simulink model "pole_placement_with_disturbance"  (R2023b)
settings: Solver=FixedStepAuto  StartTime=0.0  StopTime=Tend_slk  RelTol=1e-3
values from neighbouring files (symbols this model uses):
  A_r = [Alin M ... (first row only)    [main_pole.m]
  B_r = [Blin; zeros(3,3)]    [main_pole.m]
  C_r = [eye(6) N]    [main_pole.m]
  D_r = zeros(6,3)    [main_pole.m]
  Kv = K(:,7:9)    [main_pole.m]
  Kx = K(:,1:6)    [main_pole.m]
  L_r = place(A_r',C_r',[-50.7 -50.6 -50.5 -50.4 -50.3 -50.2 -50.1 -50 -49.9])'    [main_pole.m]
  param = [Ixx;Iyy;Izz;l;k;b;m]    [EKF_main_pole.m]    (also in main_pole.m)
  Ts_slk = 0.01    [EKF_main_pole.m]    (also in main_pole.m)
  x0 = [1;1;1;0;0;0]*(0.01)    [EKF_main_pole.m]    (also in main_pole.m = [1;1;1;0;0;0]*0.01)
libraries: SignalEditorBlockLib x1
settings Model: Creator=asus  LastModifiedBy=asus
settings OptimizationCC: ReuseModelBlockBuffer=off

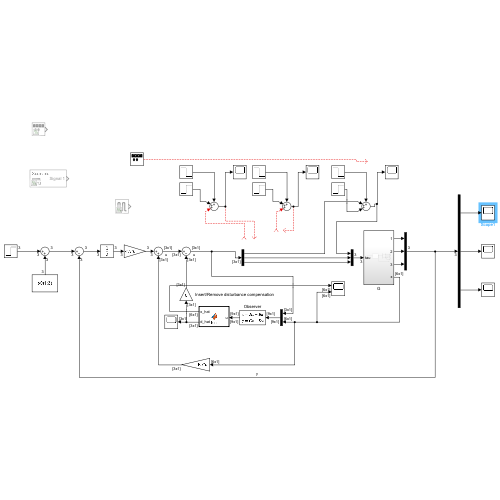
[thumbnail: Simulink's stored preview of the top-level diagram]
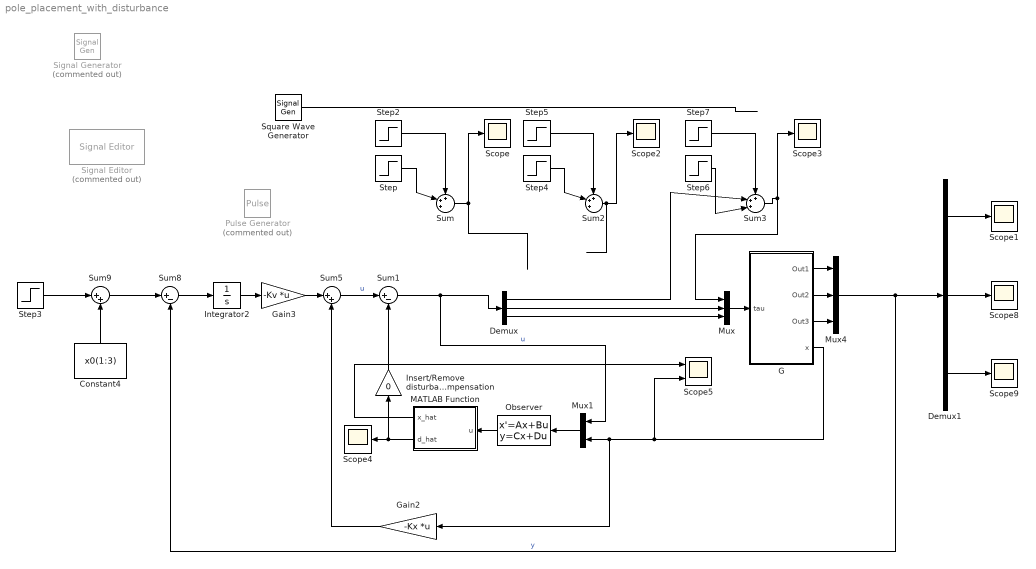
== system pole_placement_with_disturbance ==
  Constant4 : Constant  Value=x0(1:3)
  Demux : Demux  Outputs=3
  Demux1 : Demux  Outputs=3
  G : Subsystem
  Gain2 : Gain  Gain=-Kx  Multiplication=Matrix(K*u)
  Gain3 : Gain  Gain=-Kv  Multiplication=Matrix(K*u)
  Insert/Remove disturbance compensation : Gain  Gain=0
  Integrator2 : Integrator
  MATLAB Function : MATLAB Function  TreatAsAtomicUnit=on
  Mux : Mux  Inputs=3
  Mux1 : Mux  Inputs=2
  Mux4 : Mux  Inputs=3
  Observer : StateSpace  A=A_r-L_r*C_r  B=[B_r-L_r*D_r L_r]  C=eye(9)  D=zeros(9,9)  InitialCondition=0
  Pulse Generator : DiscretePulseGenerator  Commented=on  PulseType=Time based  Amplitude=0.1  Period=0.5  PulseWidth=5
  Scope{,1..4,8..9} (7 alike) : Scope
  Scope5 : Scope  NumInputPorts=2
  Signal Generator : SignalGenerator  Commented=on  WaveForm=square  Amplitude=0.1  Frequency=2  Units=rad/sec
  Signal Editor : SignalEditorBlockLib/Signal Editor  Commented=on  FileName=untitled.mat  ActiveScenario=Scenario  ActiveSignal=Signal 1  IsBus=off  OutputBusObjectStr=Bus: BusObject  SampleTime=0  Interpolate=off  ZeroCross=off  OutputAfterFinalValue=Setting to zero  Unit=inherit  PreserveSignalName=on  ApplySigPropsToAllScenarios=on  ApplySigPropsToAllSignals=off
  Square Wave Generator : SignalGenerator  WaveForm=square  Amplitude=0.1  Frequency=0.1  Units=rad/sec
  Step : Step  Time=200  After=0.1  SampleTime=Ts_slk
  Step2 : Step  Time=200.1  Before=0.1  After=0  SampleTime=Ts_slk
  Step3 : Step  Time=0  After=[0.5;0.5;0.5]*0  SampleTime=0
  Step4 : Step  Time=300  After=0.1  SampleTime=Ts_slk
  Step5 : Step  Time=300.1  Before=0.1  After=0  SampleTime=Ts_slk
  Step6 : Step  Time=350  After=0.5  SampleTime=Ts_slk
  Step7 : Step  Time=350.1  Before=0.5  After=0  SampleTime=Ts_slk
  Sum : Sum  Inputs=+++|
  Sum1 : Sum  Inputs=|+-
  Sum2 : Sum  Inputs=+++|
  Sum3 : Sum  Inputs=+++|
  Sum5 : Sum  Inputs=|++
  Sum8 : Sum  Inputs=|+-
  Sum9 : Sum  Inputs=|++
  wires:
  Mux4/1 -> Sum8/2, Demux1/1  "y"
  Sum8/1 -> Integrator2/1
  Gain2/1 -> Sum5/2
  Demux1/2 -> Scope8/1
  Gain3/1 -> Sum5/1
  Sum9/1 -> Sum8/1
  Sum1/1 -> Mux1/1, Demux/1  "u"
  Constant4/1 -> Sum9/2
  Demux1/3 -> Scope9/1
  Integrator2/1 -> Gain3/1
  Demux1/1 -> Scope1/1
  G/1(Out1) -> Mux4/1
  G/3(Out3) -> Mux4/3
  G/2(Out2) -> Mux4/2
  G/4(x) -> Scope5/2, Mux1/2, Gain2/1
  Sum/1 -> Scope/1
  ? -> Sum/3
  ? -> Sum2/3
  Mux/1 -> G/1("tau ")
  Demux/3 -> Mux/3
  Step/1 -> Sum/2
  Step2/1 -> Sum/1
  Step3/1 -> Sum9/1
  Mux1/1 -> Observer/1
  Sum5/1 -> Sum1/1  "u"
  Observer/1 -> MATLAB Function/1(u)
  Insert/Remove disturbance compensation/1 -> Sum1/2
  Step4/1 -> Sum2/2
  Sum2/1 -> Scope2/1
  Step5/1 -> Sum2/1
  Step6/1 -> Sum3/3
  Sum3/1 -> Mux/1, Scope3/1
  Step7/1 -> Sum3/1
  MATLAB Function/2(d_hat) -> Scope4/1, Insert/Remove disturbance compensation/1
  Demux/1 -> Sum3/2
  Demux/2 -> Mux/2
  Square Wave Generator/1 -> ?
  MATLAB Function/1(x_hat) -> Scope5/1

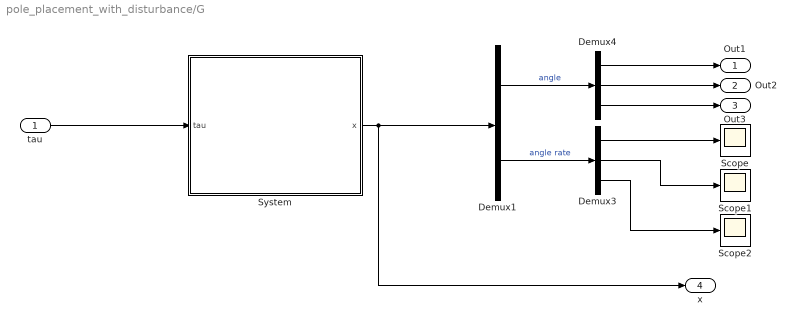
== system pole_placement_with_disturbance/G ==
  "tau " : Inport
  Demux1 : Demux  Outputs=2
  Demux3 : Demux  Outputs=3
  Demux4 : Demux  Outputs=3
  Scope : Scope
  Scope1 : Scope
  Scope2 : Scope
  System : Subsystem
  Out1 : Outport
  Out2 : Outport  Port=2
  Out3 : Outport  Port=3
  x : Outport  Port=4
  wires:
  Demux4/3 -> Out3/1
  System/1(x) -> x/1, Demux1/1
  Demux3/1 -> Scope/1
  Demux4/1 -> Out1/1
  Demux1/1 -> Demux4/1  "angle"
  Demux1/2 -> Demux3/1  "angle rate"
  Demux3/2 -> Scope1/1
  Demux4/2 -> Out2/1
  "tau "/1 -> System/1("tau ")
  Demux3/3 -> Scope2/1

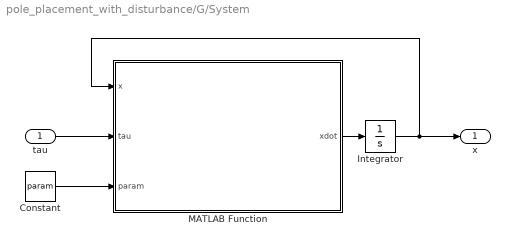
== system pole_placement_with_disturbance/G/System ==
  "tau " : Inport
  Constant : Constant  Value=param
  Integrator : Integrator  InitialCondition=x0
  MATLAB Function : MATLAB Function  TreatAsAtomicUnit=on
  x : Outport
  wires:
  Integrator/1 -> MATLAB Function/1(x), x/1
  MATLAB Function/1(xdot) -> Integrator/1
  "tau "/1 -> MATLAB Function/2(tau)
  Constant/1 -> MATLAB Function/3(param)

== matlab function pole_placement_with_disturbance/G/System/MATLAB Function ==
  data: x input; tau input; xdot output; param input
function xdot =quadcopter(x,tau,param)
% Inputs:
%           x       (model state)
%           tau     (torque)           
%           param   (model parameters)
%
% Outputs:  x_dot  (derivative of the state with respect to time)

% Parameters
g        =       9.81;           %  gravity acceleration (m/s^2)
Ixx      =       param(1,1);     %  moment of inertia 
Iyy      =       param(2,1);     %  moment of inertia
Izz      =       param(3,1);     %  moment of inertia 

% States
phi      =       x(1,1);     %  roll angle (rad)
theta    =       x(2,1);     %  pitch angle (rad)
psi      =       x(3,1);     %  yaw angle (rad)  
phi_dot  =       x(4,1);     %  roll rate (rad/s)
theta_dot=       x(5,1);     %  pitch rate (rad/s)
psi_dot  =       x(6,1);     %  yaw rate (rad/s)  

cph         =       cos(phi);
cth         =       cos(theta);
cps         =       cos(psi);
sph         =       sin(phi);
sth         =       sin(theta);
sps         =       sin(psi);

% torques
tau_1    =       tau(1,1);   %  roll torque 
tau_2    =       tau(2,1);   %  pitch torque 
tau_3    =       tau(3,1);   %  yaw torque   

% Coriolis matrix
C11=  0;
C12= (Iyy-Izz)*(theta_dot*cph*sph+psi_dot*sph^2*cth)+(Izz-Iyy)*psi_dot*cph^2*cth-Ixx*psi_dot*cth;
C13= (Izz-Iyy)*psi_dot*cph*sph*cth^2;
C21= (Izz-Iyy)*(theta_dot*cph*sph+psi_dot*sph*cth)+(Iyy-Izz)*psi_dot*cph^2*cth+Ixx*psi_dot*cth;
C22= (Izz-Iyy)*psi_dot*cph*sph;
C23= -Ixx*psi_dot*sth*cth+Iyy*psi_dot*sph^2*sth*cth+Izz*psi_dot*cph^2*sth*cth;
C31= (Iyy-Izz)*psi_dot*cth^2*sph*cph-Ixx*theta_dot*cth;
C32= (Izz-Iyy)*(theta_dot*cph*sph*sth+phi_dot*sph^2*cth)+(Iyy-Izz)*phi_dot*cph^2*cth+Ixx*psi_dot*sth*cth-Iyy*psi_dot*sph^2*sth*cth-Izz*psi_dot*cph^2*sth*cth;
C33= (Iyy-Izz)*phi_dot*cph*sph*cth^2-Iyy*theta_dot*sph^2*cth*sth-Izz*theta_dot*cph^2*cth*sth+Ixx*theta_dot*cth*sth;

C  = [C11 C12 C13;
    C21 C22 C23;
    C31 C32 C33];

% Inertia matrix
J11= Ixx;
J12= 0;
J13= -Ixx*sth;
J21= 0;
J22= Iyy*cph^2+Izz*sph^2;
J23= (Iyy-Izz)*cph*sph*cth;
J31= -Ixx*sth;
J32= (Iyy-Izz)*cph*sph*cth;
J33= Ixx*sth^2+Iyy*sph^2*cth^2+Izz*cph^2*cth^2;

J  = [J11 J12 J13;
    J21 J22 J23;
    J31 J32 J33];
v_wind = 2;
Cdz    = 0.176;
R      = 0.0125;
Az     = 4*pi*R^2;
rho    = 1.204;
Fdz    =-1/2*rho*Cdz*Az*v_wind^2*sign(v_wind);
Fd     = [0;0;Fdz];
%% Model Equation 
invJ = [ (J22*J33 - J23*J32)/(J11*J22*J33 - J11*J23*J32 - J12*J21*J33 + J12*J23*J31 + J13*J21*J32 - J13*J22*J31), -(J12*J33 - J13*J32)/(J11*J22*J33 - J11*J23*J32 - J12*J21*J33 + J12*J23*J31 + J13*J21*J32 - J13*J22*J31),  (J12*J23 - J13*J22)/(J11*J22*J33 - J11*J23*J32 - J12*J21*J33 + J12*J23*J31 + J13*J21*J32 - J13*J22*J31);
         -(J21*J33 - J23*J31)/(J11*J22*J33 - J11*J23*J32 - J12*J21*J33 + J12*J23*J31 + J13*J21*J32 - J13*J22*J31),  (J11*J33 - J13*J31)/(J11*J22*J33 - J11*J23*J32 - J12*J21*J33 + J12*J23*J31 + J13*J21*J32 - J13*J22*J31), -(J11*J23 - J13*J21)/(J11*J22*J33 - J11*J23*J32 - J12*J21*J33 + J12*J23*J31 + J13*J21*J32 - J13*J22*J31);
         (J21*J32 - J22*J31)/(J11*J22*J33 - J11*J23*J32 - J12*J21*J33 + J12*J23*J31 + J13*J21*J32 - J13*J22*J31), -(J11*J32 - J12*J31)/(J11*J22*J33 - J11*J23*J32 - J12*J21*J33 + J12*J23*J31 + J13*J21*J32 - J13*J22*J31),  (J11*J22 - J12*J21)/(J11*J22*J33 - J11*J23*J32 - J12*J21*J33 + J12*J23*J31 + J13*J21*J32 - J13*J22*J31);];

xdot        = zeros(6,1);
xdot(1:3,1) = x(4:6,1);
% xdot(4:6,1) = invJ*(tau - C*x(4:6,1));
xdot(4:6,1) = invJ*(tau - Fd - C*x(4:6,1));

== matlab function pole_placement_with_disturbance/MATLAB Function ==
  data: u input; x_hat output; d_hat output
function [x_hat,d_hat] = fcn(u)
 x_hat = u(1:6);
 d_hat = u(7:9);
